simulink model "helicopter1"  (Simulink 7.7)
settings: Solver=ode3  StartTime=0.0  StopTime=120  FixedStep=0.01  RelTol=1e-9
values from neighbouring files (symbols this model uses):
  denF = 1    [best_case.m]    (also in main.m; run_helicopter.m; utitlities.m; worst_case.m)
  denG = [1/lp 1 0]    [best_case.m]    (also in main.m = 1; run_helicopter.m; utitlities.m; worst_case.m)
  gi = .03    (= 0.03)    [best_case.m]    (also in main.m; utitlities.m = 0.05; worst_case.m)
  k = .1    (= 0.1)    [best_case.m]    (also in main.m; utitlities.m = 0.15; worst_case.m = 0.15)
  numF = 1    [best_case.m]    (also in main.m; run_helicopter.m; utitlities.m; worst_case.m)
  numG = [kd kp ki]    [best_case.m]    (also in main.m = 1; run_helicopter.m; utitlities.m; worst_case.m)
  T = .09    (= 0.09)    [best_case.m]    (also in main.m = 0.1; utitlities.m; worst_case.m = 0.11)
  wn = 1.0    (= 1)    [best_case.m]    (also in main.m; utitlities.m = 1.25; worst_case.m = 1.5)
libraries: simulink x2
settings Model: Creator=mgsanz  LastModifiedBy=Ed
settings OptimizationCC: InlineInvariantSignals=on  InitFltsAndDblsToZero=on
settings DebuggingCC: SaveWithParameterizedLinksMsg=none  SignalResolutionControl=TryResolveAllWithWarning  MultiTaskDSMMsg=warning  MultiTaskCondExecSysMsg=none  StrictBusMsg=None
settings RTWCC: IncludeERTFirstTime=on
settings GRTTargetCC: TargetFcnLib=ansi_tfl_tmw.mat

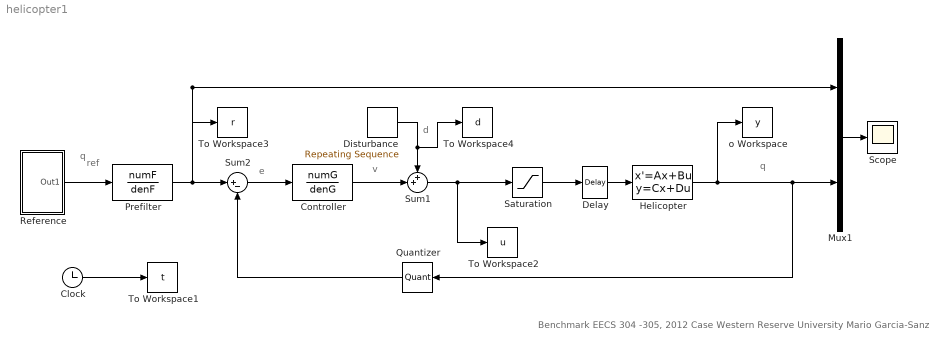
== system helicopter1 ==
  note: Benchmark EECS 304 -305, 2012
      | Case Western Reserve University
      | Mario Garcia-Sanz
  note: q
  note: q
  note: ref
  note: v
  note: e
  note: d
  Clock : Clock
      settings: Decimation=10
  Controller : TransferFcn  Numerator=numG  Denominator=denG
  Delay : TransportDelay  DelayTime=T
  Disturbance : simulink/Sources/Repeating Sequence  SystemSampleTime=-1  rep_seq_t="[0 65 65 67 67  120]"  rep_seq_y="[0  0  -17 -17   0        0]"
  Helicopter : StateSpace  A=[0 1; -wn^2 -2*gi*wn]  B=[0; k*wn^2]  C=[1 0]  D=0  X0=[-20*pi/180; 0]
  Mux1 : Mux  Inputs=2
  Prefilter : TransferFcn  Numerator=numF  Denominator=denF
  Quantizer : Quantizer  QuantizationInterval=0.0015
  Reference : Subsystem
  Saturation : Saturate  UpperLimit=2.6  LowerLimit=-17.4
  Scope : Scope
      settings: TimeRange=120  YMin=-0.4  YMax=0.3
  Sum1 : Sum  Inputs=++|
  Sum2 : Sum  Inputs=|+-
  To Workspace1 : ToWorkspace  VariableName=t  SampleTime=-1  SaveFormat=Array
  To Workspace2 : ToWorkspace  VariableName=u  SampleTime=-1  SaveFormat=Array
  To Workspace3 : ToWorkspace  VariableName=r  SampleTime=-1  SaveFormat=Array
  To Workspace4 : ToWorkspace  VariableName=d  SampleTime=-1  SaveFormat=Array
  o Workspace : ToWorkspace  VariableName=y  SampleTime=-1  SaveFormat=Array
  wires:
  Sum1/1 -> To Workspace2/1, Saturation/1
  Sum2/1 -> Controller/1
  Mux1/1 -> Scope/1
  Reference/1(Out1) -> Prefilter/1
  Clock/1 -> To Workspace1/1
  Disturbance/1 -> Sum1/1, To Workspace4/1
  Controller/1 -> Sum1/2
  Helicopter/1 -> Mux1/2, Quantizer/1, o Workspace/1
  Saturation/1 -> Delay/1
  Quantizer/1 -> Sum2/2
  Delay/1 -> Helicopter/1
  Prefilter/1 -> Sum2/1, Mux1/1, To Workspace3/1

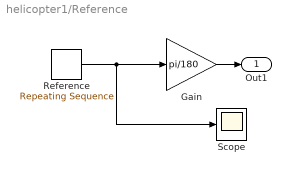
== system helicopter1/Reference ==
  Gain : Gain  Gain=pi/180
  Reference : simulink/Sources/Repeating Sequence  SystemSampleTime=-1  rep_seq_t="[0      30    50    80    80    95    97    99   101   103   105   109    113   115   120]"  rep_seq_y="[-20  -20   0   0   10  10  4.3 -0.8 -5.3 -9.2 -12.5 -17.3 -19.7     -20       -20]"
  Scope : Scope
      settings: TimeRange=120  YMin=-0.4  YMax=0.3
  Out1 : Outport
  wires:
  Reference/1 -> Gain/1, Scope/1
  Gain/1 -> Out1/1
